simulink model "model_Banks"  (R2018a)
settings: Solver=FixedStepAuto  StartTime=0  StopTime=150  FixedStep=0.1  RelTol=1e-3
settings Model: Creator=bsolv  LastModifiedBy=Jay
settings CodeAppCC: StateflowObjectComments=on

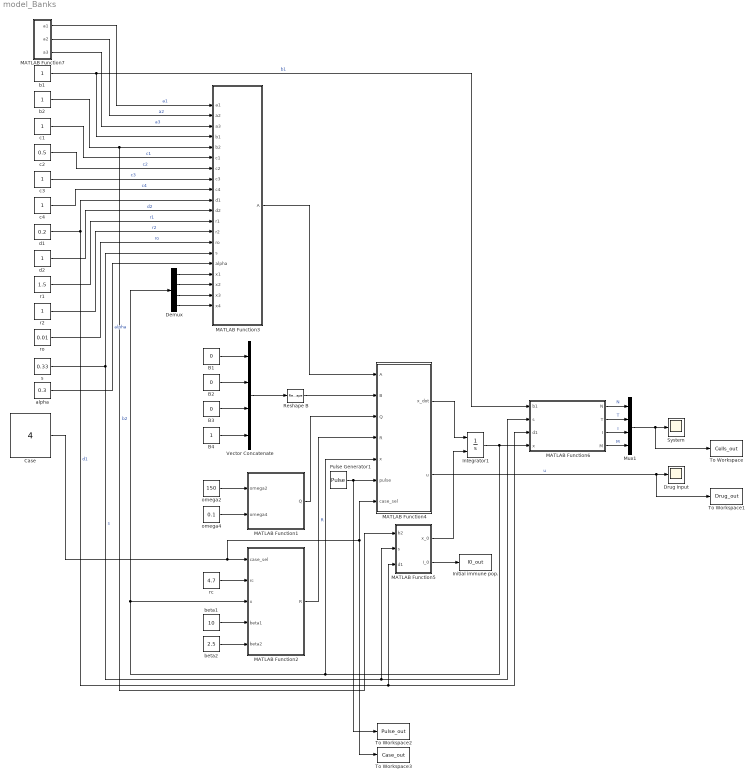
== system model_Banks ==
  B1 : Constant  Value=0
  B2 : Constant  Value=0
  B3 : Constant  Value=0
  B4 : Constant
  Case : Constant  Value=4
  Demux : Demux
  Drug Input : Scope
  Initial immune pop. : ToWorkspace  VariableName=I0_out  SaveFormat=Timeseries  SampleTime=-1
  Integrator1 : Integrator  InitialConditionSource=external  InitialCondition=[1-1;0.2;0.15-0.33/0.2;0]
  MATLAB Function1 : MATLAB Function  TreatAsAtomicUnit=on
  MATLAB Function2 : MATLAB Function  TreatAsAtomicUnit=on
  MATLAB Function3 : MATLAB Function  TreatAsAtomicUnit=on
  MATLAB Function4 : MATLAB Function  TreatAsAtomicUnit=on
  MATLAB Function5 : MATLAB Function  TreatAsAtomicUnit=on
  MATLAB Function6 : MATLAB Function  TreatAsAtomicUnit=on
  MATLAB Function7 : MATLAB Function  TreatAsAtomicUnit=on
  Mux1 : Mux
  Pulse Generator1 : DiscretePulseGenerator  Period=4  PulseWidth=3
  Reshape B : Reshape  OutputDimensionality=Column vector (2-D)
  System : Scope
  To Workspace : ToWorkspace  VariableName=Cells_out  SaveFormat=Timeseries  SampleTime=-1
  To Workspace1 : ToWorkspace  VariableName=Drug_out  SaveFormat=Timeseries  SampleTime=1
  To Workspace2 : ToWorkspace  VariableName=Pulse_out  SaveFormat=Timeseries  SampleTime=-1
  To Workspace3 : ToWorkspace  VariableName=Case_out  SaveFormat=Timeseries  SampleTime=-1
  Vector Concatenate : Concatenate  NumInputs=4
  alpha : Constant  Value=0.3
  b1 : Constant
  b2 : Constant
  beta1 : Constant  Value=10
  beta2 : Constant  Value=2.5
  c1 : Constant
  c2 : Constant  Value=0.5
  c3 : Constant
  c4 : Constant
  d1 : Constant  Value=0.2
  d2 : Constant
  omega2 : Constant  Value=150
  omega4 : Constant  Value=0.1
  r1 : Constant  Value=1.5
  r2 : Constant
  rc : Constant  Value=4.7
  ro : Constant  Value=0.01
  s : Constant  Value=0.33
  wires:
  rc/1 -> MATLAB Function2/2(rc)
  beta1/1 -> MATLAB Function2/4(beta1)
  B1/1 -> Vector Concatenate/1
  B2/1 -> Vector Concatenate/2
  B3/1 -> Vector Concatenate/3
  B4/1 -> Vector Concatenate/4
  Vector Concatenate/1 -> Reshape B/1
  MATLAB Function3/1(A) -> MATLAB Function4/1(A)
  Reshape B/1 -> MATLAB Function4/2(B)
  MATLAB Function1/1(Q) -> MATLAB Function4/3(Q)
  MATLAB Function2/1(R) -> MATLAB Function4/4(R)  "R"
  Demux/1 -> MATLAB Function3/17(x1)
  Demux/2 -> MATLAB Function3/18(x2)
  Demux/3 -> MATLAB Function3/19(x3)
  Demux/4 -> MATLAB Function3/20(x4)
  MATLAB Function7/1(a1) -> MATLAB Function3/1(a1)  "a1"
  MATLAB Function7/2(a2) -> MATLAB Function3/2(a2)  "a2"
  MATLAB Function7/3(a3) -> MATLAB Function3/3(a3)  "a3"
  b1/1 -> MATLAB Function6/1(b1), MATLAB Function3/4(b1)  "b1"
  b2/1 -> MATLAB Function3/5(b2), MATLAB Function5/1(b2)  "b2"
  c1/1 -> MATLAB Function3/6(c1)  "c1"
  c2/1 -> MATLAB Function3/7(c2)  "c2"
  c3/1 -> MATLAB Function3/8(c3)  "c3"
  c4/1 -> MATLAB Function3/9(c4)  "c4"
  d1/1 -> MATLAB Function3/10(d1), MATLAB Function5/3(d1), MATLAB Function6/3(d1)  "d1"
  d2/1 -> MATLAB Function3/11(d2)  "d2"
  r1/1 -> MATLAB Function3/12(r1)  "r1"
  r2/1 -> MATLAB Function3/13(r2)  "r2"
  s/1 -> MATLAB Function6/2(s), MATLAB Function5/2(s), MATLAB Function3/15(s)  "s"
  ro/1 -> MATLAB Function3/14(ro)  "ro"
  alpha/1 -> MATLAB Function3/16(alpha)  "alpha"
  MATLAB Function6/1(N) -> Mux1/1  "N"
  MATLAB Function6/2(T) -> Mux1/2  "T"
  MATLAB Function6/3(I) -> Mux1/3  "I"
  MATLAB Function6/4(M) -> Mux1/4  "M"
  MATLAB Function4/1(x_dot) -> Integrator1/1
  Integrator1/1 -> MATLAB Function6/4(x), MATLAB Function4/5(x), Demux/1, MATLAB Function2/3(x)
  Mux1/1 -> To Workspace/1, System/1
  MATLAB Function4/2(u) -> To Workspace1/1, Drug Input/1  "u"
  beta2/1 -> MATLAB Function2/5(beta2)
  MATLAB Function5/1(x_0) -> Integrator1/2
  Case/1 -> To Workspace3/1, MATLAB Function4/7(case_sel), MATLAB Function2/1(case_sel)
  MATLAB Function5/2(I_0) -> Initial immune pop./1
  Pulse Generator1/1 -> MATLAB Function4/6(pulse), To Workspace2/1
  omega4/1 -> MATLAB Function1/2(omega4)
  omega2/1 -> MATLAB Function1/1(omega2)

== matlab function model_Banks/MATLAB Function1 ==
  data: omega2 input; omega4 input; Q output
function Q = Q_matrix(omega2, omega4)

Q = [ 0       0       0      0;
      0       omega2  0      0; 
      0       0       0      0; 
      0       0       0      omega4];

== matlab function model_Banks/MATLAB Function7 ==
  data: a1 output; a2 output; a3 output
function [a1, a2, a3] = a()

%     de pillis
    a1 = 0.2;
    a2 = 0.3;
    a3 = 0.1;
    
%     % banks
%     a1 = 0.1;
%     a2 = 0.15;
%     a3 = 0.05;

%%% and T(0)=0.25 vs 0.20

== matlab function model_Banks/MATLAB Function2 ==
  data: case_sel input; rc input; R output; x input; beta1 input; beta2 input
function R = R_matrix(case_sel, rc, x, beta1, beta2)

x2 = x(2);
switch case_sel

    case 2
        R = rc + beta1*x2;

    case 3
        R = rc -beta2*x2;
        
    otherwise  % case 1 & 4
        R = rc;


end

== matlab function model_Banks/MATLAB Function3 ==
  data: a1 input; A output; a2 input; a3 input; b1 input; b2 input; c1 input; c2 input; c3 input; c4 input; d1 input; d2 input; r1 input; r2 input; ro input; s input; alpha input; x1 input; x2 input; x3 input; x4 input
function A = A_matrix(a1, a2, a3, b1, b2, c1, c2, c3, c4, d1, d2, r1, r2, ro, s, alpha, x1, x2, x3, x4)

    A11 =  -r2*(1+b2*x1); 
    A12 =  -c4*(x1 + 1/b2);
    A13 =  0; 
    A14 =  -a3*(1/b2 + x1);

    A21 =  -c3*x2;
    A22 =  r1*(1-b1*x2)-(c2*s/d1 + c3/b2);
    A23 =  -c2*x2;
    A24 =  -a2*x2;
        
    A31 =  0;
    A32 =  ro*(x3 + s/d1)/(alpha + x2) -c1*(x3+s/d1) -x4;
    A33 =  -d1; 
    A34 =  -a1*(x3 + s/d1)+x2;
    
    A41 =  0;
    A42 =  0;
    A43 =  0;
    A44 =  -d2;
    
    A = [A11 A12 A13 A14;
         A21 A22 A23 A24;
         A31 A32 A33 A34;
         A41 A42 A43 A44];

== matlab function model_Banks/MATLAB Function4 ==
  data: A input; B input; Q input; R input; x input; x_dot output; u output; pulse input; case_sel input
function [x_dot, u] = SDRE(A, B, Q, R, x, pulse, case_sel)

coder.extrinsic('care');

control = 1;

switch case_sel
    
    case 4
        bound = 1;
    otherwise
        bound = 0;
end

u_min = 0;
u_max = 1;
x_dot = zeros(4,1);


if(control && pulse)
    
    P = zeros(4,4);
    L = zeros(4,1);
    G = zeros(1,4);
    S = zeros(4,1);
    E = eye(4);

%     [P,~,G] = care(A,B,Q,R,S,E)
%     [P,~,~] = care(A,B,Q,R);
%     [P,~,G] = care(A,B,Q,R,S,E);
    
%     P = Riccati(A, B, Q, R);

% % % working
    P = ARE_diag(A, B, Q, R);
    G = B'/R*P;
% % %     

    u_unb = -G*x;
    if u_unb < 0
        u_unb = 0;
    end
    
    if(bound && pulse)
        u = min(max(u_unb,u_min),u_max);
    else
        u = u_unb;
    end
%     x_dot = (A-B*G)*x;
    x_dot = (A*x+B*u);
    
else
    u = 0;
    x_dot = (A)*x;
end

== matlab function model_Banks/MATLAB Function6 ==
  data: b1 input; s input; d1 input; x input; N output; T output; I output; M output
function [N, T, I, M] = DimensionaliseModel(b1, s, d1, x)

N = 0;
T = 0;
I = 0;
M = 0;

N = x(1) + 1/b1;
T = x(2);
I = x(3) + s/d1;
M = x(4);

== matlab function model_Banks/MATLAB Function5 ==
  data: x_0 output; b2 input; s input; d1 input; I_0 output
function [x_0, I_0] = init_x(b2,s,d1)

    N_0 = 1; T_0 = 0.25; I_0 = 0.15; M_0 = 0;
    
    x1_0 = N_0 - 1/b2;
    x2_0 = T_0;
    x3_0 = I_0 - s/d1;
    x4_0 = M_0;
    
    x_0 = [x1_0; x2_0; x3_0; x4_0];
